simulink model "TF_DOF1_simulink"  (R2024b)
settings: Solver=FixedStepAuto  StartTime=0.0  StopTime=10.0  FixedStep=1e-2  RelTol=1e-3
values from neighbouring files (symbols this model uses):
  A2 = [0 1;-k/m -b/m]    [TF_DOF1.m]
  b = 2    [TF_DOF1.m]
  B2 = [0; 1/m]    [TF_DOF1.m]
  C2 = eye(2,2)    [TF_DOF1.m]
  D2 = zeros(2,1)    [TF_DOF1.m]
  F0 = 1    [TF_DOF1.m]
  k = 50    [TF_DOF1.m]
  m = 1    [TF_DOF1.m]
  omega = 5    [TF_DOF1.m]
  v0 = 0    [TF_DOF1.m]
  x0 = -0.5    [TF_DOF1.m]
undefined symbols (not defined in the file or in its folder): A1, B1, C1, D1
settings Model: Creator=FK  LastModifiedBy=FK

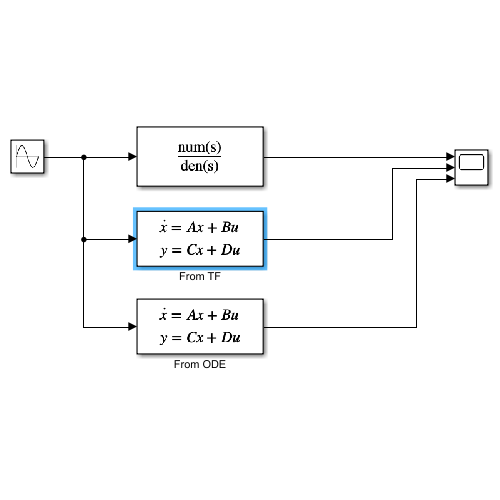
[thumbnail: Simulink's stored preview of the top-level diagram]
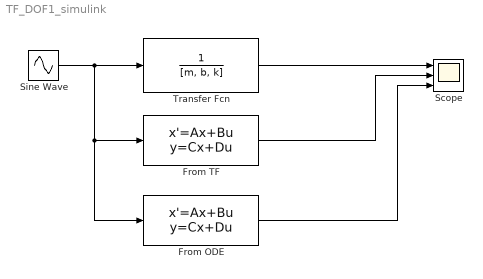
== system TF_DOF1_simulink ==
  From ODE : StateSpace  A=A2  B=B2  C=C2  D=D2  InitialCondition=[x0, v0]
  From TF : StateSpace  A=A1  B=B1  C=C1  D=D1  InitialCondition=[v0,x0]
  Scope : Scope  NumInputPorts=3
  Sine Wave : Sin  Amplitude=F0  Frequency=omega  SampleTime=0
  Transfer Fcn : TransferFcn  Denominator=[m, b, k]
  wires:
  Transfer Fcn/1 -> Scope/1
  Sine Wave/1 -> From ODE/1, From TF/1, Transfer Fcn/1
  From TF/1 -> Scope/2
  From ODE/1 -> Scope/3
